simulink model "DiscreteFirFilter_TestGen15"  (R2017b)
settings: Solver=FixedStepDiscrete  StartTime=0.0  StopTime=10.0  RelTol=1e-3
settings Model: Creator=hbourbou  LastModifiedBy=hbourbou
settings DebuggingCC: ParameterOverflowMsg=none

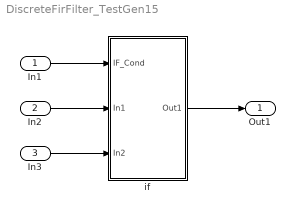
== system DiscreteFirFilter_TestGen15 ==
  In1 : Inport
  In2 : Inport  Port=2
  In3 : Inport  Port=3
  if : Subsystem  AncestorBlock=Block_TestLib/if
  Out1 : Outport
  wires:
  In1/1 -> if/1(IF_Cond)
  In2/1 -> if/2(In1)
  In3/1 -> if/3(In2)
  if/1(Out1) -> Out1/1

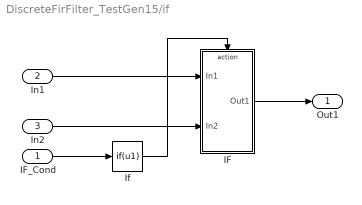
== system DiscreteFirFilter_TestGen15/if ==
  IF_Cond : Inport  OutDataTypeStr=boolean
  In1 : Inport  Port=2
  In2 : Inport  Port=3
  IF : Subsystem  TreatAsAtomicUnit=on
  If : If  IfExpression=u1  ShowElse=off
  Out1 : Outport
  wires:
  If/1 -> IF/Action
  In1/1 -> IF/1(In1)
  In2/1 -> IF/2(In2)
  IF_Cond/1 -> If/1
  IF/1(Out1) -> Out1/1

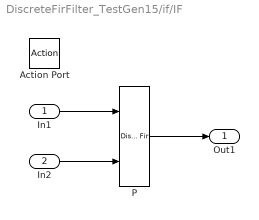
== system DiscreteFirFilter_TestGen15/if/IF ==
  In1 : Inport
  In2 : Inport  Port=2
  Action Port : ActionPort  ActionType=then
  P : DiscreteFir  CoefSource=Input port  OutDataTypeStr=int32  RndMeth=Ceiling
      settings: InputPortMap=u0,u1
  Out1 : Outport
  wires:
  In1/1 -> P/1
  In2/1 -> P/2
  P/1 -> Out1/1
